simulink library "SimscapeCustomComponents_lib"  (R2025b)
settings: Solver=VariableStepAuto  StartTime=0.0  StopTime=10.0  RelTol=1e-3
undefined symbols (not defined in the file or in its folder): base, baseVdc, capacity, DiscIntNeverNeededParam, ee_sli_rtmsupport, filterInductance, freqeuncy, frequency, gcbh, gflInverter, gfmInverter, iMaxPU, Inertia, initialSOC, plantRating, solar, Ts, ups, Vac, windSystem, windTurbine
libraries: fl_lib x397, nesl_utility x171, eeGeneralControl x85, ee_lib x82, simulink x72, datacenter_lib x68, eeTransforms x38, slpidlib x24, buildingEnergy_lib x20, SimscapeFluids_lib x17, eeSinusoidalMeasurementV2 x8, eePwmGenerator x8
(part 12 of 24)

== system SimscapeCustomComponents_lib/Datacenter/Assemblies/PDU + CDU Assembly (TL-TL)/PDU Racks (TL)/Server Tray (TL) ==
  Cold Plate : Subsystem  mask{pipeLen=pipeLen, pipeArea=pipeArea, pipeDia=pipeDia, pipeLenXtra=pipeLenXtra, thermalR=thermalKtc, initialT=initialT, initialP=initialP}
      mask prompts: pipeLen "Cold plate pipe length (m)"; pipeArea "Pipe cross-section area (m^2)"; pipeDia "Pipe hydraulic diameter (m)"; pipeLenXtra "Aggregate equivalent length of local resistances (m)"; thermalR "IT tray to cold plate thermal resistance (K/W)"; initialT "Initial temperature (K)"; initialP "Initial pressure (MPa)"
      settings: CopyFcn=set_param(gcbh,'LinkStatus','none');  PortSchema="{\"entries\":[{\"content\":{\"sides\":[{\"content\":{\"connectorIds\":[\"LConn1\"]},\"type\":\"ConnectorPlacement.EquallySpacedRectSide\",\"uuid\":\"8838d57f-01eb-4279-bd1c-25d25bcf5ace\"},{\"content\":{\"connectorIds\":[\"RConn1\"],\"side\":\"RIGHT\"},\"type\":\"ConnectorPlacement.EquallySpacedRectSide\",\"uuid\":\"56ae8252-1580-44dd-87b9-8c427bc34f49\"},{\"content\":{\"connectorIds\":[\"LConn2\"],\"side\":\"TOP\"},\"type\":\"ConnectorPlacement.EquallySpacedRectSide\",\"uuid\":\"52c6abaa-a3e9-4948-a21c-7378e8bd6fd9\"}]},\"type\":\"ConnectorPlacement.EquallySpacedConnector\",\"uuid\":\"7eb709cb-ec6a-4cc7-adbc-64cff18012b9\"}],\"packageUris\":[\"http://schema.mathworks.com/mf0/Connector/R2020b\"],\"version\":\"1.0\"}"
      mask Help: web("DocumentationColdPlate.html")
      mask DialogControl Container4 Prompt: Cold Plate
      mask DialogControl Container5 Prompt: Initial Conditions
      mask Display: image('icon_coldplate.png');
  Server Tray : Subsystem  mask{nGPU=nGPU, gpuTDPperDie=gpuTDPperDie, gpuIdlePower=gpuIdlePower, gpuHBMpower=gpuHBMpower, gpuExponent=gpuExponent, gpuHBMutil=gpuHBMutil, gpuLeakage=gpuLeakage, gpuNominalDieT=gpuLeakage, gpuDieThermalC=gpuDieThermalC, gpuHeatSinkR=gpuHeatSinkR, gpuSurfArea=gpuSurfArea, gpuAmbientR=gpuAmbientR, nCPU=nCPU, cpuTDPperSocket=cpuTDPperSocket, cpuIdlePower=cpuIdlePower, cpuExponent=cpuExponent, cpuLeakage=cpuLeakage, cpuNominalDieT=cpuNominalDieT, cpuDieThermalC=cpuDieThermalC, cpuHeatSinkR=cpuHeatSinkR, cpuSurfArea=cpuSurfArea, cpuAmbientR=cpuAmbientR, trayMass=trayMass, trayCp=trayCp, trayThermalR=trayThermalR, initialT=initialT, htc=htc}
      mask prompts: nGPU "Number of GPU (-)"; gpuTDPperDie "GPU TDP per die (W)"; gpuIdlePower "GPU idle power (W)"; gpuHBMpower "HBM power per GPU (W)"; gpuExponent "GPU power utilization exponent (-)"; gpuHBMutil "HBM utilization as fraction of compute utilization (-)"; gpuLeakage "Leakage increase per K above nominal temperature (W/K)"; gpuNominalDieT "Nominal die temperature at TDP (K)"; gpuDieThermalC "GPU die thermal capacitance (J/K)"; gpuHeatSinkR "GPU die-heat-sink thermal resistance (K/W)"; gpuSurfArea "Surface area per die for ambient heat transfer (m^2)"; gpuAmbientR "GPU die-ambient thermal resistance (K/W)"; nCPU "Number of CPU (-)"; cpuTDPperSocket "CPU TDP per socket (W)"; cpuIdlePower "CPU idle power per socket (W)"; cpuExponent "CPU power utilization exponent (-)"; cpuLeakage "Leakage increase per K above nominal temperature (W/K)"; cpuNominalDieT "Nominal die temperature at TDP (K)"; cpuDieThermalC "CPU die thermal capacitance (J/K)"; cpuHeatSinkR "CPU die-heat-sink thermal resistance (K/W)"; cpuSurfArea "Surface area per die for ambient heat transfer (m^2)"; cpuAmbientR "CPU die-ambient thermal resistance (K/W)"; trayMass "Tray mass (kg)"; trayCp "Tray specific heat capacity (J/kg*K)"; trayThermalR "Tray to external thermal resistance (K/W)"; initialT "Initial temperature (K)"; htc "Heat transfer coefficient to ambient (W/m^2.K)"
      settings: CopyFcn=set_param(gcbh,'LinkStatus','none');  PortSchema="{\"entries\":[{\"content\":{\"sides\":[{\"content\":{\"connectorIds\":[\"LConn1\",\"LConn2\",\"LConn3\"]},\"type\":\"ConnectorPlacement.EquallySpacedRectSide\",\"uuid\":\"893f21b9-92d6-433a-96e5-f8193a696c29\"},{\"content\":{\"connectorIds\":[\"RConn1\",\"RConn2\",\"RConn3\"],\"side\":\"RIGHT\"},\"type\":\"ConnectorPlacement.EquallySpacedRectSide\",\"uuid\":\"efd10409-70d8-4a6a-97a2-13f0e6f538e3\"},{\"content\":{\"side\":\"TOP\"},\"type\":\"ConnectorPlacement.EquallySpacedRectSide\",\"uuid\":\"8c9765cd-90e6-46de-916c-606bbb93143e\"},{\"content\":{\"connectorIds\":[\"RConn4\"],\"side\":\"BOTTOM\"},\"type\":\"ConnectorPlacement.EquallySpacedRectSide\",\"uuid\":\"9656b44e-d582-43b0-a7fe-c629821d6c27\"}]},\"type\":\"ConnectorPlacement.EquallySpacedConnector\",\"uuid\":\"add7a682-eb4b-4f46-a5b9-e161ccf96de5\"}],\"packageUris\":[\"http://schema.mathworks.com/mf0/Connector/R2020b\"],\"version\":\"1.0\"}"
      mask Help: web("DocumentationServerTray.html")
      mask DialogControl Container6 Prompt: GPU
      mask DialogControl Container7 Prompt: CPU
      mask DialogControl Container9 Prompt: IT Tray
      mask DialogControl Container8 Prompt: Initial Conditions
      mask Display: image('icon_serverPlate.png');
  U_gpu : PMIOPort  Side=Left
  U_cpu : PMIOPort  Port=2  Side=Left
  Ha : PMIOPort  Port=3  Side=Left
  P : PMIOPort  Port=4  Side=Right
  T_gpu : PMIOPort  Port=5  Side=Right
  T_cpu : PMIOPort  Port=6  Side=Right
  A : PMIOPort  Port=7  Side=Right
  B : PMIOPort  Port=8  Side=Right
  connections:
  Server Tray/RConn2 -- T_gpu/RConn1
  Server Tray/RConn3 -- T_cpu/RConn1
  Server Tray/RConn1 -- P/RConn1
  Cold Plate/RConn1 -- B/RConn1
  Cold Plate/LConn1 -- A/RConn1
  Server Tray/LConn2 -- U_cpu/RConn1
  Server Tray/LConn1 -- U_gpu/RConn1
  Server Tray/LConn3 -- Ha/RConn1
  Cold Plate/LConn2 -- Server Tray/RConn4

== system SimscapeCustomComponents_lib/Datacenter/Facilities/Solid State Transformer/Converters/Subsystem1 ==
  PhA : Inport
  ma : Inport  Port=2
  Array Connection : SimscapeArrayConnection  NumScalarElements=3
  Array Connection1 : SimscapeArrayConnection  NumScalarElements=3
  CHB Phase Leg (Average Model) : datacenter_lib/CHB Phase Leg (Average Model)  NumModules=3  OnResistance=1e-3 Ohm  InitialDCVoltage=4400 V  GridVoltage=13800 V  TotalDCVoltage=13200 V
      settings: InternalSimscapePortConfiguration="{\"Bottom\":[],\"Left\":[{\"id\":\"ACPositive\",\"label\":\"AC+\",\"type\":\"foundation.electrical.electrical\"},{\"id\":\"ACNegative\",\"label\":\"AC-\",\"type\":\"foundation.electrical.electrical\"},{\"id\":\"m\",\"label\":\"m\",\"type\":\"input\"}],\"Right\":[{\"id\":\"DCPositive\",\"label\":\"DC+\",\"type\":\"foundation.electrical.electrical\"},{\"id\":\"DCNegative\",\"label\":\"DC-\",\"type\":\"foundation.electrical.electrical\"}],\"Top\":[]}"
  Capacitor : fl_lib/Electrical/Electrical Elements/Capacitor  c=0.005 F  r=1e-6 Ohm  g=0 1/Ohm  i_specify=off  i_priority=None  i=0 A  i_nominal_specify=off  i_nominal_value=1  i_nominal_unit=A  v_specify=off  v_priority=None  v=0 V  v_nominal_specify=off  v_nominal_value=1  v_nominal_unit=V  vc_specify=on  vc_priority=None  vc=4400 V  vc_nominal_specify=off  vc_nominal_value=1  vc_nominal_unit=V
  Capacitor1 : fl_lib/Electrical/Electrical Elements/Capacitor  c=0.005 F  r=1e-6 Ohm  g=0 1/Ohm  i_specify=off  i_priority=None  i=0 A  i_nominal_specify=off  i_nominal_value=1  i_nominal_unit=A  v_specify=off  v_priority=None  v=0 V  v_nominal_specify=off  v_nominal_value=1  v_nominal_unit=V  vc_specify=on  vc_priority=None  vc=4400 V  vc_nominal_specify=off  vc_nominal_value=1  vc_nominal_unit=V
  Capacitor2 : fl_lib/Electrical/Electrical Elements/Capacitor  c=0.005 F  r=1e-6 Ohm  g=0 1/Ohm  i_specify=off  i_priority=None  i=0 A  i_nominal_specify=off  i_nominal_value=1  i_nominal_unit=A  v_specify=off  v_priority=None  v=0 V  v_nominal_specify=off  v_nominal_value=1  v_nominal_unit=V  vc_specify=on  vc_priority=None  vc=4400 V  vc_nominal_specify=off  vc_nominal_value=1  vc_nominal_unit=V
  DAB Generalized Average Model : datacenter_lib/DAB Generalized Average Model  N=5.5  L1=3.4e-05 H  L2=1.12e-06 H  Rt=0.005 Ohm  Co=0.001 F  fs=20000 Hz  vo0_init=800 V  it1R_init=0 A  it1I_init=0 A  include_esr=false  Rc=0.25 Ohm  i_in_specify=on  i_in_priority=None  i_in=0 A  i_in_nominal_specify=off  i_in_nominal_value=1  i_in_nominal_unit=A  i_out_specify=on  i_out_priority=None  i_out=0 A  i_out_nominal_specify=off  i_out_nominal_value=1  i_out_nominal_unit=A  v_in_specify=on  v_in_priority=None  v_in=0 V  v_in_nominal_specify=off  v_in_nominal_value=1  v_in_nominal_unit=V  v_out_specify=on  v_out_priority=None  v_out=0 V  v_out_nominal_specify=off  v_out_nominal_value=1  v_out_nominal_unit=V
      settings: InternalSimscapePortConfiguration="{\"Bottom\":[],\"Left\":[{\"id\":\"p_in\",\"label\":\"V+\",\"type\":\"foundation.electrical.electrical\"},{\"id\":\"n_in\",\"label\":\"V-\",\"type\":\"foundation.electrical.electrical\"},{\"id\":\"d\",\"label\":\"d\",\"type\":\"input\"}],\"Right\":[{\"id\":\"p_out\",\"label\":\"Vo+\",\"type\":\"foundation.electrical.electrical\"},{\"id\":\"n_out\",\"label\":\"Vo-\",\"type\":\"foundation.electrical.electrical\"}],\"Top\":[]}"
  DAB Generalized Average Model1 : datacenter_lib/DAB Generalized Average Model  N=5.5  L1=3.4e-05 H  L2=1.12e-06 H  Rt=0.005 Ohm  Co=0.001 F  fs=20000 Hz  vo0_init=800 V  it1R_init=0 A  it1I_init=0 A  include_esr=false  Rc=0.25 Ohm  i_in_specify=on  i_in_priority=None  i_in=0 A  i_in_nominal_specify=off  i_in_nominal_value=1  i_in_nominal_unit=A  i_out_specify=on  i_out_priority=None  i_out=0 A  i_out_nominal_specify=off  i_out_nominal_value=1  i_out_nominal_unit=A  v_in_specify=on  v_in_priority=None  v_in=0 V  v_in_nominal_specify=off  v_in_nominal_value=1  v_in_nominal_unit=V  v_out_specify=on  v_out_priority=None  v_out=0 V  v_out_nominal_specify=off  v_out_nominal_value=1  v_out_nominal_unit=V
      settings: InternalSimscapePortConfiguration="{\"Bottom\":[],\"Left\":[{\"id\":\"p_in\",\"label\":\"V+\",\"type\":\"foundation.electrical.electrical\"},{\"id\":\"n_in\",\"label\":\"V-\",\"type\":\"foundation.electrical.electrical\"},{\"id\":\"d\",\"label\":\"d\",\"type\":\"input\"}],\"Right\":[{\"id\":\"p_out\",\"label\":\"Vo+\",\"type\":\"foundation.electrical.electrical\"},{\"id\":\"n_out\",\"label\":\"Vo-\",\"type\":\"foundation.electrical.electrical\"}],\"Top\":[]}"
  DAB Generalized Average Model2 : datacenter_lib/DAB Generalized Average Model  N=5.5  L1=3.4e-05 H  L2=1.12e-06 H  Rt=0.005 Ohm  Co=0.001 F  fs=20000 Hz  vo0_init=800 V  it1R_init=0 A  it1I_init=0 A  include_esr=false  Rc=0.25 Ohm  i_in_specify=on  i_in_priority=None  i_in=0 A  i_in_nominal_specify=off  i_in_nominal_value=1  i_in_nominal_unit=A  i_out_specify=on  i_out_priority=None  i_out=0 A  i_out_nominal_specify=off  i_out_nominal_value=1  i_out_nominal_unit=A  v_in_specify=on  v_in_priority=None  v_in=0 V  v_in_nominal_specify=off  v_in_nominal_value=1  v_in_nominal_unit=V  v_out_specify=on  v_out_priority=None  v_out=0 V  v_out_nominal_specify=off  v_out_nominal_value=1  v_out_nominal_unit=V
      settings: InternalSimscapePortConfiguration="{\"Bottom\":[],\"Left\":[{\"id\":\"p_in\",\"label\":\"V+\",\"type\":\"foundation.electrical.electrical\"},{\"id\":\"n_in\",\"label\":\"V-\",\"type\":\"foundation.electrical.electrical\"},{\"id\":\"d\",\"label\":\"d\",\"type\":\"input\"}],\"Right\":[{\"id\":\"p_out\",\"label\":\"Vo+\",\"type\":\"foundation.electrical.electrical\"},{\"id\":\"n_out\",\"label\":\"Vo-\",\"type\":\"foundation.electrical.electrical\"}],\"Top\":[]}"
  Delay : Delay  DelayLength=1
  Delay1 : Delay  DelayLength=1  InitialCondition=1
  Electrical Reference : fl_lib/Electrical/Electrical Elements/Electrical Reference
  Gain : Gain  Gain=1/dcOutputVoltage
  Low-Pass Filter (Discrete or Continuous) : eeGeneralControl/Low-Pass Filter (Discrete or Continuous)  K=1  T=0.005  B=inf  A=-inf  init_option=Inherited from block input  x0=0  Ts=-1
  PS-Simulink Converter : nesl_utility/PS-Simulink Converter  PhysicalDomain=network_engine_domain  SubClassName=ps_output  LeftPortType=input  RightPortType=output  PseudoPeriodic=off  Frequencies=[]  VectorFormat=inherit  Unit=inherit  AffineConversion=off
  PS-Simulink Converter1 : nesl_utility/PS-Simulink Converter  PhysicalDomain=network_engine_domain  SubClassName=ps_output  LeftPortType=input  RightPortType=output  PseudoPeriodic=off  Frequencies=[]  VectorFormat=inherit  Unit=inherit  AffineConversion=off
  Simulink-PS Converter : nesl_utility/Simulink-PS Converter  PhysicalDomain=network_engine_domain  SubClassName=ps_input  LeftPortType=input  RightPortType=output  PseudoPeriodic=off  Frequencies=[]  NoiseDistribution=none  NoiseParameters=[]  Unit=1  AffineConversion=off  FilteringAndDerivatives=provide  SimscapeFilterOrder=1  InputFilterTimeConstant=0.001  UdotUserProvided=0
  Simulink-PS Converter1 : nesl_utility/Simulink-PS Converter  PhysicalDomain=network_engine_domain  SubClassName=ps_input  LeftPortType=input  RightPortType=output  PseudoPeriodic=off  Frequencies=[]  NoiseDistribution=none  NoiseParameters=[]  Unit=1  AffineConversion=off  FilteringAndDerivatives=provide  SimscapeFilterOrder=1  InputFilterTimeConstant=0.001  UdotUserProvided=0
  Voltage Sensor : fl_lib/Electrical/Electrical Sensors/Voltage Sensor
  Voltage Sensor1 : fl_lib/Electrical/Electrical Sensors/Voltage Sensor
  AC + : PMIOPort  Side=Left
  AC - : PMIOPort  Port=2  Side=Left
  + : PMIOPort  Port=3  Side=Right
  - : PMIOPort  Port=4  Side=Right
  Out1 : Outport
  V_out_pu : Outport  Port=2
  wires:
  PS-Simulink Converter/1 -> Delay/1
  Delay/1 -> Low-Pass Filter (Discrete or Continuous)/1
  Low-Pass Filter (Discrete or Continuous)/1 -> Out1/1
  PS-Simulink Converter1/1 -> Delay1/1
  Delay1/1 -> Gain/1
  PhA/1 -> Simulink-PS Converter/1
  Gain/1 -> V_out_pu/1
  ma/1 -> Simulink-PS Converter1/1
  connections:
  PS-Simulink Converter/LConn1 -- Voltage Sensor/RConn1
  DAB Generalized Average Model1/LConn1 -- Array Connection/LConn2 -- Capacitor1/LConn1
  DAB Generalized Average Model1/LConn2 -- Array Connection1/LConn2 -- Capacitor1/RConn1
  Voltage Sensor/LConn1 -- Array Connection/LConn1 -- Capacitor/LConn1 -- DAB Generalized Average Model/LConn1
  CHB Phase Leg (Average Model)/LConn1 -- AC +/RConn1
  DAB Generalized Average Model2/LConn2 -- Array Connection1/LConn3 -- Capacitor2/RConn1
  DAB Generalized Average Model2/LConn1 -- Array Connection/LConn3 -- Capacitor2/LConn1
  CHB Phase Leg (Average Model)/LConn2 -- AC -/RConn1
  Voltage Sensor/RConn2 -- Capacitor/RConn1 -- Array Connection1/LConn1 -- DAB Generalized Average Model/LConn2
  +/RConn1 -- Voltage Sensor1/LConn1 -- DAB Generalized Average Model2/RConn1 -- DAB Generalized Average Model1/RConn1 -- DAB Generalized Average Model/RConn1
  -/RConn1 -- Electrical Reference/LConn1 -- Voltage Sensor1/RConn2 -- DAB Generalized Average Model/RConn2 -- DAB Generalized Average Model2/RConn2 -- DAB Generalized Average Model1/RConn2
  PS-Simulink Converter1/LConn1 -- Voltage Sensor1/RConn1
  Simulink-PS Converter/RConn1 -- DAB Generalized Average Model2/LConn3 -- DAB Generalized Average Model1/LConn3 -- DAB Generalized Average Model/LConn3
  Array Connection/RConn1 -- CHB Phase Leg (Average Model)/RConn1
  Array Connection1/RConn1 -- CHB Phase Leg (Average Model)/RConn2
  Simulink-PS Converter1/RConn1 -- CHB Phase Leg (Average Model)/LConn3

== system SimscapeCustomComponents_lib/Datacenter/Facilities/Solid State Transformer/Converters/Subsystem2 ==
  PhB : Inport
  mb : Inport  Port=2
  Array Connection : SimscapeArrayConnection  NumScalarElements=3
  Array Connection1 : SimscapeArrayConnection  NumScalarElements=3
  CHB Phase Leg (Average Model) : datacenter_lib/CHB Phase Leg (Average Model)  NumModules=3  OnResistance=1e-3 Ohm  InitialDCVoltage=4400 V  GridVoltage=13800 V  TotalDCVoltage=13200 V
      settings: InternalSimscapePortConfiguration="{\"Bottom\":[],\"Left\":[{\"id\":\"ACPositive\",\"label\":\"AC+\",\"type\":\"foundation.electrical.electrical\"},{\"id\":\"ACNegative\",\"label\":\"AC-\",\"type\":\"foundation.electrical.electrical\"},{\"id\":\"m\",\"label\":\"m\",\"type\":\"input\"}],\"Right\":[{\"id\":\"DCPositive\",\"label\":\"DC+\",\"type\":\"foundation.electrical.electrical\"},{\"id\":\"DCNegative\",\"label\":\"DC-\",\"type\":\"foundation.electrical.electrical\"}],\"Top\":[]}"
  Capacitor : fl_lib/Electrical/Electrical Elements/Capacitor  c=0.005 F  r=1e-6 Ohm  g=0 1/Ohm  i_specify=off  i_priority=None  i=0 A  i_nominal_specify=off  i_nominal_value=1  i_nominal_unit=A  v_specify=off  v_priority=None  v=0 V  v_nominal_specify=off  v_nominal_value=1  v_nominal_unit=V  vc_specify=on  vc_priority=None  vc=4400 V  vc_nominal_specify=off  vc_nominal_value=1  vc_nominal_unit=V
  Capacitor1 : fl_lib/Electrical/Electrical Elements/Capacitor  c=0.005 F  r=1e-6 Ohm  g=0 1/Ohm  i_specify=off  i_priority=None  i=0 A  i_nominal_specify=off  i_nominal_value=1  i_nominal_unit=A  v_specify=off  v_priority=None  v=0 V  v_nominal_specify=off  v_nominal_value=1  v_nominal_unit=V  vc_specify=on  vc_priority=None  vc=4400 V  vc_nominal_specify=off  vc_nominal_value=1  vc_nominal_unit=V
  Capacitor2 : fl_lib/Electrical/Electrical Elements/Capacitor  c=0.005 F  r=1e-6 Ohm  g=0 1/Ohm  i_specify=off  i_priority=None  i=0 A  i_nominal_specify=off  i_nominal_value=1  i_nominal_unit=A  v_specify=off  v_priority=None  v=0 V  v_nominal_specify=off  v_nominal_value=1  v_nominal_unit=V  vc_specify=on  vc_priority=None  vc=4400 V  vc_nominal_specify=off  vc_nominal_value=1  vc_nominal_unit=V
  DAB Generalized Average Model : datacenter_lib/DAB Generalized Average Model  N=5.5  L1=3.4e-05 H  L2=1.12e-06 H  Rt=0.005 Ohm  Co=0.001 F  fs=20000 Hz  vo0_init=800 V  it1R_init=0 A  it1I_init=0 A  include_esr=false  Rc=0.25 Ohm  i_in_specify=on  i_in_priority=None  i_in=0 A  i_in_nominal_specify=off  i_in_nominal_value=1  i_in_nominal_unit=A  i_out_specify=on  i_out_priority=None  i_out=0 A  i_out_nominal_specify=off  i_out_nominal_value=1  i_out_nominal_unit=A  v_in_specify=on  v_in_priority=None  v_in=0 V  v_in_nominal_specify=off  v_in_nominal_value=1  v_in_nominal_unit=V  v_out_specify=on  v_out_priority=None  v_out=0 V  v_out_nominal_specify=off  v_out_nominal_value=1  v_out_nominal_unit=V
      settings: InternalSimscapePortConfiguration="{\"Bottom\":[],\"Left\":[{\"id\":\"p_in\",\"label\":\"V+\",\"type\":\"foundation.electrical.electrical\"},{\"id\":\"n_in\",\"label\":\"V-\",\"type\":\"foundation.electrical.electrical\"},{\"id\":\"d\",\"label\":\"d\",\"type\":\"input\"}],\"Right\":[{\"id\":\"p_out\",\"label\":\"Vo+\",\"type\":\"foundation.electrical.electrical\"},{\"id\":\"n_out\",\"label\":\"Vo-\",\"type\":\"foundation.electrical.electrical\"}],\"Top\":[]}"
  DAB Generalized Average Model1 : datacenter_lib/DAB Generalized Average Model  N=5.5  L1=3.4e-05 H  L2=1.12e-06 H  Rt=0.005 Ohm  Co=0.001 F  fs=20000 Hz  vo0_init=800 V  it1R_init=0 A  it1I_init=0 A  include_esr=false  Rc=0.25 Ohm  i_in_specify=on  i_in_priority=None  i_in=0 A  i_in_nominal_specify=off  i_in_nominal_value=1  i_in_nominal_unit=A  i_out_specify=on  i_out_priority=None  i_out=0 A  i_out_nominal_specify=off  i_out_nominal_value=1  i_out_nominal_unit=A  v_in_specify=on  v_in_priority=None  v_in=0 V  v_in_nominal_specify=off  v_in_nominal_value=1  v_in_nominal_unit=V  v_out_specify=on  v_out_priority=None  v_out=0 V  v_out_nominal_specify=off  v_out_nominal_value=1  v_out_nominal_unit=V
      settings: InternalSimscapePortConfiguration="{\"Bottom\":[],\"Left\":[{\"id\":\"p_in\",\"label\":\"V+\",\"type\":\"foundation.electrical.electrical\"},{\"id\":\"n_in\",\"label\":\"V-\",\"type\":\"foundation.electrical.electrical\"},{\"id\":\"d\",\"label\":\"d\",\"type\":\"input\"}],\"Right\":[{\"id\":\"p_out\",\"label\":\"Vo+\",\"type\":\"foundation.electrical.electrical\"},{\"id\":\"n_out\",\"label\":\"Vo-\",\"type\":\"foundation.electrical.electrical\"}],\"Top\":[]}"
  DAB Generalized Average Model2 : datacenter_lib/DAB Generalized Average Model  N=5.5  L1=3.4e-05 H  L2=1.12e-06 H  Rt=0.005 Ohm  Co=0.001 F  fs=20000 Hz  vo0_init=800 V  it1R_init=0 A  it1I_init=0 A  include_esr=false  Rc=0.25 Ohm  i_in_specify=on  i_in_priority=None  i_in=0 A  i_in_nominal_specify=off  i_in_nominal_value=1  i_in_nominal_unit=A  i_out_specify=on  i_out_priority=None  i_out=0 A  i_out_nominal_specify=off  i_out_nominal_value=1  i_out_nominal_unit=A  v_in_specify=on  v_in_priority=None  v_in=0 V  v_in_nominal_specify=off  v_in_nominal_value=1  v_in_nominal_unit=V  v_out_specify=on  v_out_priority=None  v_out=0 V  v_out_nominal_specify=off  v_out_nominal_value=1  v_out_nominal_unit=V
      settings: InternalSimscapePortConfiguration="{\"Bottom\":[],\"Left\":[{\"id\":\"p_in\",\"label\":\"V+\",\"type\":\"foundation.electrical.electrical\"},{\"id\":\"n_in\",\"label\":\"V-\",\"type\":\"foundation.electrical.electrical\"},{\"id\":\"d\",\"label\":\"d\",\"type\":\"input\"}],\"Right\":[{\"id\":\"p_out\",\"label\":\"Vo+\",\"type\":\"foundation.electrical.electrical\"},{\"id\":\"n_out\",\"label\":\"Vo-\",\"type\":\"foundation.electrical.electrical\"}],\"Top\":[]}"
  Delay : Delay  DelayLength=1
  Delay1 : Delay  DelayLength=1  InitialCondition=1
  Electrical Reference : fl_lib/Electrical/Electrical Elements/Electrical Reference
  Gain : Gain  Gain=1/dcOutputVoltage
  Low-Pass Filter (Discrete or Continuous) : eeGeneralControl/Low-Pass Filter (Discrete or Continuous)  K=1  T=0.005  B=inf  A=-inf  init_option=Inherited from block input  x0=0  Ts=-1
  PS-Simulink Converter : nesl_utility/PS-Simulink Converter  PhysicalDomain=network_engine_domain  SubClassName=ps_output  LeftPortType=input  RightPortType=output  PseudoPeriodic=off  Frequencies=[]  VectorFormat=inherit  Unit=inherit  AffineConversion=off
  PS-Simulink Converter1 : nesl_utility/PS-Simulink Converter  PhysicalDomain=network_engine_domain  SubClassName=ps_output  LeftPortType=input  RightPortType=output  PseudoPeriodic=off  Frequencies=[]  VectorFormat=inherit  Unit=inherit  AffineConversion=off
  Scope : Scope
      settings: ActiveDisplayYMinimum=-1  ActiveDisplayYMaximum=1
  Simulink-PS Converter : nesl_utility/Simulink-PS Converter  PhysicalDomain=network_engine_domain  SubClassName=ps_input  LeftPortType=input  RightPortType=output  PseudoPeriodic=off  Frequencies=[]  NoiseDistribution=none  NoiseParameters=[]  Unit=1  AffineConversion=off  FilteringAndDerivatives=provide  SimscapeFilterOrder=1  InputFilterTimeConstant=0.001  UdotUserProvided=0
  Simulink-PS Converter1 : nesl_utility/Simulink-PS Converter  PhysicalDomain=network_engine_domain  SubClassName=ps_input  LeftPortType=input  RightPortType=output  PseudoPeriodic=off  Frequencies=[]  NoiseDistribution=none  NoiseParameters=[]  Unit=1  AffineConversion=off  FilteringAndDerivatives=provide  SimscapeFilterOrder=1  InputFilterTimeConstant=0.001  UdotUserProvided=0
  Voltage Sensor : fl_lib/Electrical/Electrical Sensors/Voltage Sensor
  Voltage Sensor1 : fl_lib/Electrical/Electrical Sensors/Voltage Sensor
  AC + : PMIOPort  Side=Left
  AC - : PMIOPort  Port=2  Side=Left
  + : PMIOPort  Port=3  Side=Right
  - : PMIOPort  Port=4  Side=Right
  Out1 : Outport
  V_out_pu : Outport  Port=2
  wires:
  PS-Simulink Converter/1 -> Delay/1, Scope/1
  Delay/1 -> Low-Pass Filter (Discrete or Continuous)/1
  Low-Pass Filter (Discrete or Continuous)/1 -> Out1/1
  PS-Simulink Converter1/1 -> Delay1/1
  Delay1/1 -> Gain/1
  PhB/1 -> Simulink-PS Converter/1
  Gain/1 -> V_out_pu/1
  mb/1 -> Simulink-PS Converter1/1
  connections:
  PS-Simulink Converter/LConn1 -- Voltage Sensor/RConn1
  DAB Generalized Average Model1/LConn1 -- Capacitor1/LConn1 -- Array Connection/LConn2
  Capacitor1/RConn1 -- DAB Generalized Average Model1/LConn2 -- Array Connection1/LConn2
  Capacitor/LConn1 -- Voltage Sensor/LConn1 -- DAB Generalized Average Model/LConn1 -- Array Connection/LConn1
  CHB Phase Leg (Average Model)/LConn1 -- AC +/RConn1
  DAB Generalized Average Model2/LConn2 -- Capacitor2/RConn1 -- Array Connection1/LConn3
  Capacitor2/LConn1 -- DAB Generalized Average Model2/LConn1 -- Array Connection/LConn3
  CHB Phase Leg (Average Model)/LConn2 -- AC -/RConn1
  Array Connection1/LConn1 -- Voltage Sensor/RConn2 -- DAB Generalized Average Model/LConn2 -- Capacitor/RConn1
  +/RConn1 -- Voltage Sensor1/LConn1 -- DAB Generalized Average Model2/RConn1 -- DAB Generalized Average Model1/RConn1 -- DAB Generalized Average Model/RConn1
  -/RConn1 -- Electrical Reference/LConn1 -- Voltage Sensor1/RConn2 -- DAB Generalized Average Model/RConn2 -- DAB Generalized Average Model2/RConn2 -- DAB Generalized Average Model1/RConn2
  PS-Simulink Converter1/LConn1 -- Voltage Sensor1/RConn1
  Simulink-PS Converter/RConn1 -- DAB Generalized Average Model2/LConn3 -- DAB Generalized Average Model1/LConn3 -- DAB Generalized Average Model/LConn3
  Array Connection/RConn1 -- CHB Phase Leg (Average Model)/RConn1
  Array Connection1/RConn1 -- CHB Phase Leg (Average Model)/RConn2
  CHB Phase Leg (Average Model)/LConn3 -- Simulink-PS Converter1/RConn1

== system SimscapeCustomComponents_lib/Datacenter/Facilities/Solid State Transformer/Converters/Subsystem3 ==
  PhC : Inport
  mc : Inport  Port=2
  Array Connection : SimscapeArrayConnection  NumScalarElements=3
  Array Connection1 : SimscapeArrayConnection  NumScalarElements=3
  CHB Phase Leg (Average Model) : datacenter_lib/CHB Phase Leg (Average Model)  NumModules=3  OnResistance=1e-3 Ohm  InitialDCVoltage=4400 V  GridVoltage=13800 V  TotalDCVoltage=13200 V
      settings: InternalSimscapePortConfiguration="{\"Bottom\":[],\"Left\":[{\"id\":\"ACPositive\",\"label\":\"AC+\",\"type\":\"foundation.electrical.electrical\"},{\"id\":\"ACNegative\",\"label\":\"AC-\",\"type\":\"foundation.electrical.electrical\"},{\"id\":\"m\",\"label\":\"m\",\"type\":\"input\"}],\"Right\":[{\"id\":\"DCPositive\",\"label\":\"DC+\",\"type\":\"foundation.electrical.electrical\"},{\"id\":\"DCNegative\",\"label\":\"DC-\",\"type\":\"foundation.electrical.electrical\"}],\"Top\":[]}"
  Capacitor : fl_lib/Electrical/Electrical Elements/Capacitor  c=0.005 F  r=1e-6 Ohm  g=0 1/Ohm  i_specify=off  i_priority=None  i=0 A  i_nominal_specify=off  i_nominal_value=1  i_nominal_unit=A  v_specify=off  v_priority=None  v=0 V  v_nominal_specify=off  v_nominal_value=1  v_nominal_unit=V  vc_specify=on  vc_priority=None  vc=4400 V  vc_nominal_specify=off  vc_nominal_value=1  vc_nominal_unit=V
  Capacitor1 : fl_lib/Electrical/Electrical Elements/Capacitor  c=0.005 F  r=1e-6 Ohm  g=0 1/Ohm  i_specify=off  i_priority=None  i=0 A  i_nominal_specify=off  i_nominal_value=1  i_nominal_unit=A  v_specify=off  v_priority=None  v=0 V  v_nominal_specify=off  v_nominal_value=1  v_nominal_unit=V  vc_specify=on  vc_priority=None  vc=4400 V  vc_nominal_specify=off  vc_nominal_value=1  vc_nominal_unit=V
  Capacitor2 : fl_lib/Electrical/Electrical Elements/Capacitor  c=0.005 F  r=1e-6 Ohm  g=0 1/Ohm  i_specify=off  i_priority=None  i=0 A  i_nominal_specify=off  i_nominal_value=1  i_nominal_unit=A  v_specify=off  v_priority=None  v=0 V  v_nominal_specify=off  v_nominal_value=1  v_nominal_unit=V  vc_specify=on  vc_priority=None  vc=4400 V  vc_nominal_specify=off  vc_nominal_value=1  vc_nominal_unit=V
  DAB Generalized Average Model : datacenter_lib/DAB Generalized Average Model  N=5.5  L1=3.4e-05 H  L2=1.12e-06 H  Rt=0.005 Ohm  Co=0.001 F  fs=20000 Hz  vo0_init=800 V  it1R_init=0 A  it1I_init=0 A  include_esr=false  Rc=0.25 Ohm  i_in_specify=on  i_in_priority=None  i_in=0 A  i_in_nominal_specify=off  i_in_nominal_value=1  i_in_nominal_unit=A  i_out_specify=on  i_out_priority=None  i_out=0 A  i_out_nominal_specify=off  i_out_nominal_value=1  i_out_nominal_unit=A  v_in_specify=on  v_in_priority=None  v_in=0 V  v_in_nominal_specify=off  v_in_nominal_value=1  v_in_nominal_unit=V  v_out_specify=on  v_out_priority=None  v_out=0 V  v_out_nominal_specify=off  v_out_nominal_value=1  v_out_nominal_unit=V
      settings: InternalSimscapePortConfiguration="{\"Bottom\":[],\"Left\":[{\"id\":\"p_in\",\"label\":\"V+\",\"type\":\"foundation.electrical.electrical\"},{\"id\":\"n_in\",\"label\":\"V-\",\"type\":\"foundation.electrical.electrical\"},{\"id\":\"d\",\"label\":\"d\",\"type\":\"input\"}],\"Right\":[{\"id\":\"p_out\",\"label\":\"Vo+\",\"type\":\"foundation.electrical.electrical\"},{\"id\":\"n_out\",\"label\":\"Vo-\",\"type\":\"foundation.electrical.electrical\"}],\"Top\":[]}"
  DAB Generalized Average Model1 : datacenter_lib/DAB Generalized Average Model  N=5.5  L1=3.4e-05 H  L2=1.12e-06 H  Rt=0.005 Ohm  Co=0.001 F  fs=20000 Hz  vo0_init=800 V  it1R_init=0 A  it1I_init=0 A  include_esr=false  Rc=0.25 Ohm  i_in_specify=on  i_in_priority=None  i_in=0 A  i_in_nominal_specify=off  i_in_nominal_value=1  i_in_nominal_unit=A  i_out_specify=on  i_out_priority=None  i_out=0 A  i_out_nominal_specify=off  i_out_nominal_value=1  i_out_nominal_unit=A  v_in_specify=on  v_in_priority=None  v_in=0 V  v_in_nominal_specify=off  v_in_nominal_value=1  v_in_nominal_unit=V  v_out_specify=on  v_out_priority=None  v_out=0 V  v_out_nominal_specify=off  v_out_nominal_value=1  v_out_nominal_unit=V
      settings: InternalSimscapePortConfiguration="{\"Bottom\":[],\"Left\":[{\"id\":\"p_in\",\"label\":\"V+\",\"type\":\"foundation.electrical.electrical\"},{\"id\":\"n_in\",\"label\":\"V-\",\"type\":\"foundation.electrical.electrical\"},{\"id\":\"d\",\"label\":\"d\",\"type\":\"input\"}],\"Right\":[{\"id\":\"p_out\",\"label\":\"Vo+\",\"type\":\"foundation.electrical.electrical\"},{\"id\":\"n_out\",\"label\":\"Vo-\",\"type\":\"foundation.electrical.electrical\"}],\"Top\":[]}"
  DAB Generalized Average Model2 : datacenter_lib/DAB Generalized Average Model  N=5.5  L1=3.4e-05 H  L2=1.12e-06 H  Rt=0.005 Ohm  Co=0.001 F  fs=20000 Hz  vo0_init=800 V  it1R_init=0 A  it1I_init=0 A  include_esr=false  Rc=0.25 Ohm  i_in_specify=on  i_in_priority=None  i_in=0 A  i_in_nominal_specify=off  i_in_nominal_value=1  i_in_nominal_unit=A  i_out_specify=on  i_out_priority=None  i_out=0 A  i_out_nominal_specify=off  i_out_nominal_value=1  i_out_nominal_unit=A  v_in_specify=on  v_in_priority=None  v_in=0 V  v_in_nominal_specify=off  v_in_nominal_value=1  v_in_nominal_unit=V  v_out_specify=on  v_out_priority=None  v_out=0 V  v_out_nominal_specify=off  v_out_nominal_value=1  v_out_nominal_unit=V
      settings: InternalSimscapePortConfiguration="{\"Bottom\":[],\"Left\":[{\"id\":\"p_in\",\"label\":\"V+\",\"type\":\"foundation.electrical.electrical\"},{\"id\":\"n_in\",\"label\":\"V-\",\"type\":\"foundation.electrical.electrical\"},{\"id\":\"d\",\"label\":\"d\",\"type\":\"input\"}],\"Right\":[{\"id\":\"p_out\",\"label\":\"Vo+\",\"type\":\"foundation.electrical.electrical\"},{\"id\":\"n_out\",\"label\":\"Vo-\",\"type\":\"foundation.electrical.electrical\"}],\"Top\":[]}"
  Delay : Delay  DelayLength=1
  Delay1 : Delay  DelayLength=1  InitialCondition=1
  Electrical Reference : fl_lib/Electrical/Electrical Elements/Electrical Reference
  Gain : Gain  Gain=1/dcOutputVoltage
  Low-Pass Filter (Discrete or Continuous) : eeGeneralControl/Low-Pass Filter (Discrete or Continuous)  K=1  T=0.005  B=inf  A=-inf  init_option=Inherited from block input  x0=0  Ts=-1
  PS-Simulink Converter : nesl_utility/PS-Simulink Converter  PhysicalDomain=network_engine_domain  SubClassName=ps_output  LeftPortType=input  RightPortType=output  PseudoPeriodic=off  Frequencies=[]  VectorFormat=inherit  Unit=inherit  AffineConversion=off
  PS-Simulink Converter1 : nesl_utility/PS-Simulink Converter  PhysicalDomain=network_engine_domain  SubClassName=ps_output  LeftPortType=input  RightPortType=output  PseudoPeriodic=off  Frequencies=[]  VectorFormat=inherit  Unit=inherit  AffineConversion=off
  Simulink-PS Converter : nesl_utility/Simulink-PS Converter  PhysicalDomain=network_engine_domain  SubClassName=ps_input  LeftPortType=input  RightPortType=output  PseudoPeriodic=off  Frequencies=[]  NoiseDistribution=none  NoiseParameters=[]  Unit=1  AffineConversion=off  FilteringAndDerivatives=provide  SimscapeFilterOrder=1  InputFilterTimeConstant=0.001  UdotUserProvided=0
  Simulink-PS Converter1 : nesl_utility/Simulink-PS Converter  PhysicalDomain=network_engine_domain  SubClassName=ps_input  LeftPortType=input  RightPortType=output  PseudoPeriodic=off  Frequencies=[]  NoiseDistribution=none  NoiseParameters=[]  Unit=1  AffineConversion=off  FilteringAndDerivatives=provide  SimscapeFilterOrder=1  InputFilterTimeConstant=0.001  UdotUserProvided=0
  Voltage Sensor : fl_lib/Electrical/Electrical Sensors/Voltage Sensor
  Voltage Sensor1 : fl_lib/Electrical/Electrical Sensors/Voltage Sensor
  AC + : PMIOPort  Side=Left
  AC - : PMIOPort  Port=2  Side=Left
  + : PMIOPort  Port=3  Side=Right
  - : PMIOPort  Port=4  Side=Right
  Out1 : Outport
  V_out_pu : Outport  Port=2
  wires:
  PS-Simulink Converter/1 -> Delay/1
  Delay/1 -> Low-Pass Filter (Discrete or Continuous)/1
  Low-Pass Filter (Discrete or Continuous)/1 -> Out1/1
  PS-Simulink Converter1/1 -> Delay1/1
  Delay1/1 -> Gain/1
  PhC/1 -> Simulink-PS Converter/1
  Gain/1 -> V_out_pu/1
  mc/1 -> Simulink-PS Converter1/1
  connections:
  PS-Simulink Converter/LConn1 -- Voltage Sensor/RConn1
  DAB Generalized Average Model1/LConn1 -- Capacitor1/LConn1 -- Array Connection/LConn2
  Capacitor1/RConn1 -- DAB Generalized Average Model1/LConn2 -- Array Connection1/LConn2
  Capacitor/LConn1 -- Voltage Sensor/LConn1 -- DAB Generalized Average Model/LConn1 -- Array Connection/LConn1
  CHB Phase Leg (Average Model)/LConn1 -- AC +/RConn1
  DAB Generalized Average Model2/LConn2 -- Capacitor2/RConn1 -- Array Connection1/LConn3
  Capacitor2/LConn1 -- DAB Generalized Average Model2/LConn1 -- Array Connection/LConn3
  CHB Phase Leg (Average Model)/LConn2 -- AC -/RConn1
  Array Connection1/LConn1 -- Voltage Sensor/RConn2 -- DAB Generalized Average Model/LConn2 -- Capacitor/RConn1
  +/RConn1 -- Voltage Sensor1/LConn1 -- DAB Generalized Average Model2/RConn1 -- DAB Generalized Average Model1/RConn1 -- DAB Generalized Average Model/RConn1
  -/RConn1 -- Electrical Reference/LConn1 -- Voltage Sensor1/RConn2 -- DAB Generalized Average Model/RConn2 -- DAB Generalized Average Model2/RConn2 -- DAB Generalized Average Model1/RConn2
  PS-Simulink Converter1/LConn1 -- Voltage Sensor1/RConn1
  Simulink-PS Converter/RConn1 -- DAB Generalized Average Model2/LConn3 -- DAB Generalized Average Model1/LConn3 -- DAB Generalized Average Model/LConn3
  Array Connection/RConn1 -- CHB Phase Leg (Average Model)/RConn1
  Array Connection1/RConn1 -- CHB Phase Leg (Average Model)/RConn2
  CHB Phase Leg (Average Model)/LConn3 -- Simulink-PS Converter1/RConn1

== system SimscapeCustomComponents_lib/Datacenter/Facilities/Solid State Transformer/DAB Controller/DAB Balancing ==
  Vdc_A : Inport
  Vdc_B : Inport  Port=2
  Vdc_C : Inport  Port=3
  Vdc_avg : Inport  Port=4
  Kbal_dab_A : Gain  Gain=0.0005
  Kbal_dab_B : Gain  Gain=0.0005
  Kbal_dab_C : Gain  Gain=0.0005
  LPF_A : DiscreteTransferFcn  Numerator=0.0018831801790618607  Denominator=[1, -0.9981168198209381]
  LPF_B : DiscreteTransferFcn  Numerator=0.0018831801790618607  Denominator=[1, -0.9981168198209381]
  LPF_C : DiscreteTransferFcn  Numerator=0.0018831801790618607  Denominator=[1, -0.9981168198209381]
  Sat_A : Saturate  UpperLimit=0.02  LowerLimit=-0.02
  Sat_B : Saturate  UpperLimit=0.02  LowerLimit=-0.02
  Sat_C : Saturate  UpperLimit=0.02  LowerLimit=-0.02
  Sub_A : Sum  Inputs=+-
  Sub_B : Sum  Inputs=+-
  Sub_C : Sum  Inputs=+-
  ZOH_A : ZeroOrderHold  SampleTime=2e-3
  ZOH_B : ZeroOrderHold  SampleTime=2e-3
  ZOH_C : ZeroOrderHold  SampleTime=2e-3
  delta_d_A : Outport
  delta_d_B : Outport  Port=2
  delta_d_C : Outport  Port=3
  wires:
  Vdc_A/1 -> Sub_A/1
  Vdc_avg/1 -> Sub_C/2, Sub_B/2, Sub_A/2
  Vdc_B/1 -> Sub_B/1
  Vdc_C/1 -> Sub_C/1
  Sub_A/1 -> ZOH_A/1
  Kbal_dab_A/1 -> Sat_A/1
  Sat_A/1 -> delta_d_A/1
  Sub_B/1 -> ZOH_B/1
  Kbal_dab_B/1 -> Sat_B/1
  Sat_B/1 -> delta_d_B/1
  Sub_C/1 -> ZOH_C/1
  Kbal_dab_C/1 -> Sat_C/1
  Sat_C/1 -> delta_d_C/1
  ZOH_A/1 -> LPF_A/1
  LPF_A/1 -> Kbal_dab_A/1
  ZOH_B/1 -> LPF_B/1
  LPF_B/1 -> Kbal_dab_B/1
  ZOH_C/1 -> LPF_C/1
  LPF_C/1 -> Kbal_dab_C/1

== system SimscapeCustomComponents_lib/Datacenter/Facilities/Solid State Transformer/Filter & AC measurements/Current ==
  Isabc : Inport
  Demux : Demux  Outputs=3
  Mux : Mux  Inputs=3
  Unit Delay : UnitDelay  SampleTime=-1
  Iabc : Outport
  wires:
  Mux/1 -> Iabc/1
  Unit Delay/1 -> Demux/1
  Isabc/1 -> Unit Delay/1
  Demux/1 -> Mux/1
  Demux/2 -> Mux/2
  Demux/3 -> Mux/3

== system SimscapeCustomComponents_lib/Datacenter/Facilities/Solid State Transformer/Filter & AC measurements/PLL ==
  Iabc : Inport
  V : Inport  Port=2
  Constant1 : Constant  Value=pi/2  SampleTime=Ts
  Data Type Conversion Inherited : simulink/Signal Attributes/Data Type Conversion Inherited  ConvertRealWorld=Real World Value  DoSatur=off
  Demux : Demux  Outputs=3
  Park Transform : eeTransforms/Park Transform  AxisAlignment=D-axis  PowerInvariant=off
  "Sinusoidal Measurement (PLL, Three-Phase)" : eeSinusoidalMeasurementV2/Sinusoidal Measurement (PLL, Three-Phase)  InputFilter=on  InputNormalization=off  Kp_LF=ups.AFE.kpPLL  Ki_LF=ups.AFE.kiPLL  F0=frequency  Theta0=0  Ts=Ts
  Sum : Sum  Inputs=|+-
  Terminator : Terminator
  Terminator2 : Terminator
  Id : Outport
  freq : Outport  Port=2
  mag : Outport  Port=3
  wires:
  Data Type Conversion Inherited/1 -> Sum/2
  Constant1/1 -> Data Type Conversion Inherited/2
  V/1 -> "Sinusoidal Measurement (PLL, Three-Phase)"/1
  "Sinusoidal Measurement (PLL, Three-Phase)"/2 -> Sum/1, Data Type Conversion Inherited/1
  Park Transform/1 -> Demux/1
  Demux/3 -> Terminator/1
  Sum/1 -> Park Transform/2
  Demux/1 -> Id/1
  "Sinusoidal Measurement (PLL, Three-Phase)"/1 -> freq/1
  Iabc/1 -> Park Transform/1
  Demux/2 -> Terminator2/1
  "Sinusoidal Measurement (PLL, Three-Phase)"/3 -> mag/1

== system SimscapeCustomComponents_lib/Datacenter/Facilities/Solid State Transformer/Filter & AC measurements/Voltage ==
  Vsabc : Inport
  Demux1 : Demux  Outputs=3
  Mux1 : Mux  Inputs=3
  Unit Delay : UnitDelay  SampleTime=-1
  Vabc : Outport
  wires:
  Mux1/1 -> Vabc/1
  Unit Delay/1 -> Demux1/1
  Vsabc/1 -> Unit Delay/1
  Demux1/1 -> Mux1/1
  Demux1/2 -> Mux1/2
  Demux1/3 -> Mux1/3

== system SimscapeCustomComponents_lib/Datacenter/Facilities/Solid State Transformer/PFC Rectifier Controller/Current Controller ==
  idRef : Inport
  iqRef : Inport  Port=2
  theta : Inport  Port=3
  vd : Inport  Port=4
  vq : Inport  Port=5
  iabc(PU) : Inport  Port=6
  Vmag : Inport  Port=7
  Reset : Inport  Port=8
  Demux1 : Demux  Outputs=3
  Id and Iq Controller : Subsystem
  Inverse Park Transform : eeTransforms/Inverse Park Transform  AxisAlignment=D-axis  PowerInvariant=off
  Park Transform : eeTransforms/Park Transform  AxisAlignment=D-axis  PowerInvariant=off
  Saturation : Saturate  UpperLimit=1.5  LowerLimit=-1.5
  Terminator1 : Terminator
  vabcRef : Outport
  IdCntrlError : Outport  Port=2
  IqCntrlError : Outport  Port=3
  Flag : Outport  Port=4
  wires:
  Id and Iq Controller/2(IdCntrlError) -> IdCntrlError/1
  Id and Iq Controller/3(IqCntrlError) -> IqCntrlError/1
  Id and Iq Controller/1(vdqoRef) -> Inverse Park Transform/1
  vq/1 -> Id and Iq Controller/6(vq)
  Demux1/2 -> Id and Iq Controller/4(iqSens)  "iqSens"
  iqRef/1 -> Id and Iq Controller/2(iqRef)
  Demux1/1 -> Id and Iq Controller/3(IdSens)  "IdSens"
  idRef/1 -> Id and Iq Controller/1(idRef)
  vd/1 -> Id and Iq Controller/5(vd)
  Inverse Park Transform/1 -> Saturation/1
  iabc(PU)/1 -> Park Transform/1
  theta/1 -> Park Transform/2, Inverse Park Transform/2
  Demux1/3 -> Terminator1/1
  Park Transform/1 -> Demux1/1
  Saturation/1 -> vabcRef/1
  Reset/1 -> Id and Iq Controller/7(Reset)
  Vmag/1 -> Id and Iq Controller/8(Vmag)
  Id and Iq Controller/4(Flag) -> Flag/1

== system SimscapeCustomComponents_lib/Datacenter/Facilities/Solid State Transformer/PFC Rectifier Controller/DC Voltage Controller and Current Reference ==
  qRef : Inport
  vPeak : Inport  Port=2
  vdcRef : Inport  Port=3
  VdcSens : Inport  Port=4
  Reset : Inport  Port=5
  Constant : Constant  SampleTime=Ts
  Data Type Conversion Inherited : simulink/Signal Attributes/Data Type Conversion Inherited  ConvertRealWorld=Real World Value  DoSatur=off
  Gain : Gain  Gain=-1
  Iq Reference : Subsystem
  Switch : Switch  Criteria=u2 > Threshold  SaturateOnIntegerOverflow=off  InputSameDT=off
  Voltage Controller : Subsystem
  idRef : Outport
  iqRef : Outport  Port=2
  wires:
  Constant/1 -> Data Type Conversion Inherited/2
  Data Type Conversion Inherited/1 -> Switch/3
  Gain/1 -> iqRef/1
  qRef/1 -> Iq Reference/2(Q_ref)
  Voltage Controller/1(Id) -> idRef/1
  vdcRef/1 -> Voltage Controller/1(Vdcref)
  VdcSens/1 -> Voltage Controller/2(Vdcmeas)
  Iq Reference/1(iq_ref) -> Gain/1
  vPeak/1 -> Switch/2, Switch/1, Data Type Conversion Inherited/1
  Switch/1 -> Iq Reference/1(V_mag)
  Reset/1 -> Voltage Controller/3(Reset)

== system SimscapeCustomComponents_lib/Datacenter/Facilities/Solid State Transformer/PFC Rectifier Controller/PLL ==
  V : Inport
  Constant1 : Constant  Value=pi/2  SampleTime=Ts
  Data Type Conversion Inherited : simulink/Signal Attributes/Data Type Conversion Inherited  ConvertRealWorld=Real World Value  DoSatur=off
  Demux : Demux  Outputs=3
  Filtered Derivative (Discrete or Continuous) : eeGeneralControl/Filtered Derivative (Discrete or Continuous)  K=1  T=0.005  B=inf  A=-inf  minRatio=10  init_option=Inherited from block input  x0=0  Ts=-1
      settings: LibrarySourceBlock=|
      | ee_sl_lib/General Control/Filtered Derivative
      | (Discrete or Continuous)
  Park Transform : eeTransforms/Park Transform  AxisAlignment=D-axis  PowerInvariant=off
  Scope : Scope  NumInputPorts=2
      settings: ActiveDisplayYMinimum=-0.12536761024201581  ActiveDisplayYMaximum=1.1283084921781426  DataLoggingVariableName=ScopeData20
  Scope1 : Scope
      settings: ActiveDisplayYMinimum=-1  ActiveDisplayYMaximum=1  DataLoggingVariableName=ScopeData21
  "Sinusoidal Measurement (PLL, Three-Phase)" : eeSinusoidalMeasurementV2/Sinusoidal Measurement (PLL, Three-Phase)  InputFilter=on  InputNormalization=off  Kp_LF=KpPLL  Ki_LF=KiPLL  F0=Freq  Theta0=0  Ts=Ts
  Sum : Sum  Inputs=|+-
  Terminator : Terminator
  Terminator1 : Terminator
  theta : Outport
  Vd : Outport  Port=2
  Vq : Outport  Port=3
  mag : Outport  Port=4
  wires:
  Data Type Conversion Inherited/1 -> Sum/2
  Constant1/1 -> Data Type Conversion Inherited/2
  V/1 -> Park Transform/1, "Sinusoidal Measurement (PLL, Three-Phase)"/1
  "Sinusoidal Measurement (PLL, Three-Phase)"/2 -> Sum/1, Data Type Conversion Inherited/1
  Park Transform/1 -> Demux/1
  Demux/3 -> Terminator/1
  "Sinusoidal Measurement (PLL, Three-Phase)"/3 -> Scope/1, mag/1
  Sum/1 -> Park Transform/2, theta/1
  Demux/2 -> Vq/1
  Demux/1 -> Scope/2, Filtered Derivative (Discrete or Continuous)/1, Vd/1
  "Sinusoidal Measurement (PLL, Three-Phase)"/1 -> Terminator1/1
  Filtered Derivative (Discrete or Continuous)/1 -> Scope1/1

== system SimscapeCustomComponents_lib/Datacenter/Facilities/Solid State Transformer/PFC Rectifier Controller/Reset Controller ==
  u : Inport
  AND : Logic  IconShape=distinctive  AllPortsSameDT=off  OutDataTypeStr=boolean
  AND1 : Logic  IconShape=distinctive  AllPortsSameDT=off  OutDataTypeStr=boolean
  Compare To Constant : simulink/Logic and Bit Operations/Compare To Constant  relop=<=  const=0.5  OutDataTypeStr=boolean
  Compare To Constant1 : simulink/Logic and Bit Operations/Compare To Constant  relop=>  const=0.5  OutDataTypeStr=boolean
  Compare To Constant2 : simulink/Logic and Bit Operations/Compare To Constant  relop=>  const=0.05  OutDataTypeStr=boolean
  Data Type Conversion : DataTypeConversion  SaturateOnIntegerOverflow=off  RndMeth=Floor
  Data Type Conversion1 : DataTypeConversion  OutDataTypeStr=double  SaturateOnIntegerOverflow=off  RndMeth=Floor
  Delay : Delay  DelayLength=1
  Discrete-Time Integrator : DiscreteIntegrator  IntegratorMethod=Integration: Backward Euler  ExternalReset=falling  SampleTime=ups.sampleTime  LimitOutput=on  UpperSaturationLimit=0.6  LowerSaturationLimit=0  ICPrevOutput=DiscIntNeverNeededParam  ICPrevScaledInput=DiscIntNeverNeededParam
  NOT : Logic  Operator=NOT  IconShape=distinctive  AllPortsSameDT=off  OutDataTypeStr=boolean
  S-R Flip-Flop : simulink_extras/Flip Flops/S-R Flip-Flop  initial_condition=0
  Scope2 : Scope
      settings: ActiveDisplayYMinimum=-0.12499999999999997  ActiveDisplayYMaximum=1.125  DataLoggingVariableName=ScopeData8
  Out1 : Outport
  wires:
  u/1 -> Compare To Constant1/1, Delay/1
  Compare To Constant1/1 -> Data Type Conversion1/1, AND/2
  Compare To Constant/1 -> AND/1
  Discrete-Time Integrator/1 -> Compare To Constant2/1
  Data Type Conversion1/1 -> Discrete-Time Integrator/2, Discrete-Time Integrator/1, AND1/1
  Delay/1 -> Compare To Constant/1
  S-R Flip-Flop/1 -> NOT/1
  AND1/1 -> Data Type Conversion/1
  AND/1 -> Scope2/1, S-R Flip-Flop/1
  Compare To Constant2/1 -> AND1/2
  Data Type Conversion/1 -> S-R Flip-Flop/2
  NOT/1 -> Out1/1

== system SimscapeCustomComponents_lib/Datacenter/PDU/PDU Racks (TL)/Server Tray (TL)/Cold Plate ==
  Pipe (TL) : fl_lib/Thermal Liquid/Elements/Pipe (TL)  length=pipeLen m  area=pipeArea m^2  Dh=pipeDia m  length_add=pipeLenXtra m  roughness=15e-6 m  Re_lam=2000  Re_tur=4000  shape_factor=64  Nu_lam=3.66  dynamic_compressibility=true  inertia=false  p0=initialP MPa  T0=initialT K  mdot0=0 kg/s  p_nominal=0.101325 MPa  T_nominal=293.15 K
  Thermal Resistance : fl_lib/Thermal/Thermal Elements/Thermal Resistance  resistance=thermalR K/W  T_specify=off  T_priority=None  T=0 K  T_nominal_specify=off  T_nominal_value=1  T_nominal_unit=K  Q_specify=off  Q_priority=None  Q=0 W  Q_nominal_specify=off  Q_nominal_value=1  Q_nominal_unit=W
  A : PMIOPort  Side=Left
  H : PMIOPort  Port=2  Side=Left
  B : PMIOPort  Port=3  Side=Right
  connections:
  Thermal Resistance/LConn1 -- H/RConn1
  Thermal Resistance/RConn1 -- Pipe (TL)/LConn2
  Pipe (TL)/LConn1 -- A/RConn1
  Pipe (TL)/RConn1 -- B/RConn1
